simulink model "cordic_test"  (R2020a)
settings: Solver=VariableStepAuto  StartTime=0.0  StopTime=2048*2048  RelTol=1e-3
libraries: library x11, simulink x5, hdlsllib x3, simulink_extras x1
settings Model: SimulationMode=rapid-accelerator  Creator=david  LastModifiedBy=david

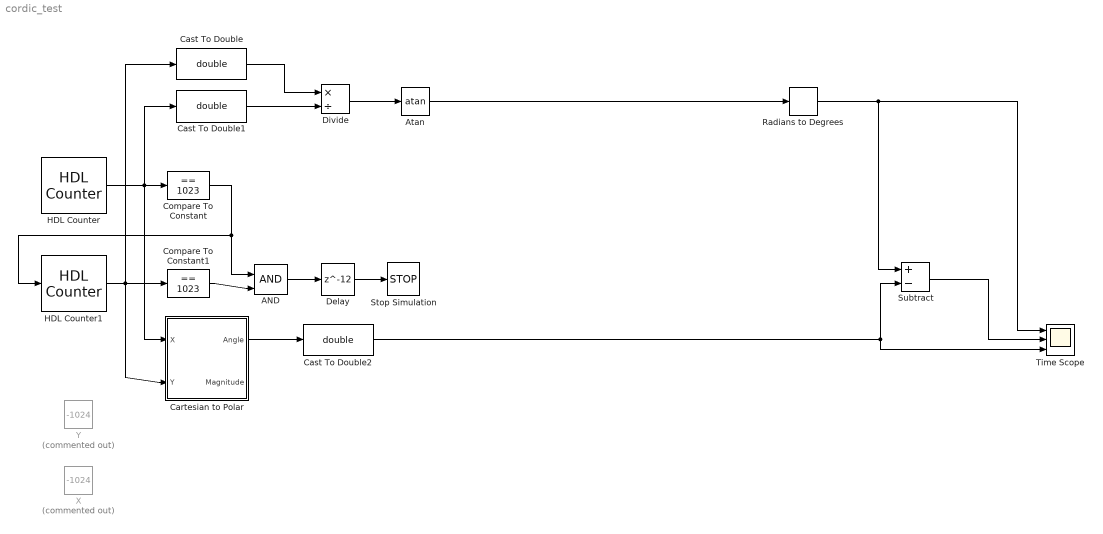
== system cordic_test ==
  AND : Logic  IconShape=distinctive  AllPortsSameDT=off  OutDataTypeStr=boolean
  Atan : Trigonometry  Operator=atan
  Cartesian to Polar : Subsystem  mask{b=16, f=8}
      mask prompts: b "Angle Wordlength:"; f "Angle Fractional Bits:"
      mask DialogControl DescGroupVar Prompt: Cartesian to Polar
      mask DialogControl DescTextVar Prompt: Convert cartesian coordinates to polar representation. This block uses Circular CORDIC operating in vectoring mode. The output angle is in the range [-90, 90] degrees.
      mask DialogControl ParameterGroupVar Prompt: Main
  Cast To Double : DataTypeConversion  OutDataTypeStr=double
  Cast To Double1 : DataTypeConversion  OutDataTypeStr=double
  Cast To Double2 : DataTypeConversion  OutDataTypeStr=double
  Compare To Constant : simulink/Logic and Bit Operations/Compare To Constant  relop===  const=1023  OutDataTypeStr=boolean
  Compare To Constant1 : simulink/Logic and Bit Operations/Compare To Constant  relop===  const=1023  OutDataTypeStr=boolean
  Delay : Delay  DelayLength=12
  Divide : Product  Inputs=*/
  HDL Counter : hdlsllib/Sources/HDL Counter  CountType=Count limited  CountInit=-1024  CountStep=1  CountMax=1023  CountFromType=Initial value  CountFrom=-1024  CountResetPort=off  CountLoadPort=off  CountEnbPort=off  CountDirPort=off  CountDataType=Signed  CountWordLen=24  CountFracLen=11  CountSampTime=1
  HDL Counter1 : hdlsllib/Sources/HDL Counter  CountType=Count limited  CountInit=-1024  CountStep=1  CountMax=1023  CountFromType=Initial value  CountFrom=-1024  CountResetPort=off  CountLoadPort=off  CountEnbPort=on  CountDirPort=off  CountDataType=Signed  CountWordLen=24  CountFracLen=11  CountSampTime=1
  Radians to Degrees : simulink_extras/Transformations/Radians to Degrees
  Stop Simulation : Stop
  Subtract : Sum  Inputs=+-
  Time Scope : Scope  NumInputPorts=3
  X : Constant  Commented=on  Value=-1024  OutDataTypeStr=fixdt(1,16,3)  SampleTime=1
  Y : Constant  Commented=on  Value=-1024  OutDataTypeStr=fixdt(1,16,3)  SampleTime=1
  wires:
  HDL Counter/1 -> Cartesian to Polar/1(X), Cast To Double1/1, Compare To Constant/1
  Compare To Constant/1 -> AND/1, HDL Counter1/1
  Divide/1 -> Atan/1
  HDL Counter1/1 -> Cartesian to Polar/2(Y), Cast To Double/1, Compare To Constant1/1
  Compare To Constant1/1 -> AND/2
  AND/1 -> Delay/1
  Delay/1 -> Stop Simulation/1
  Cast To Double/1 -> Divide/1
  Cast To Double1/1 -> Divide/2
  Atan/1 -> Radians to Degrees/1
  Radians to Degrees/1 -> Subtract/1, Time Scope/1
  Cast To Double2/1 -> Time Scope/3, Subtract/2
  Subtract/1 -> Time Scope/2
  Cartesian to Polar/1(Angle) -> Cast To Double2/1

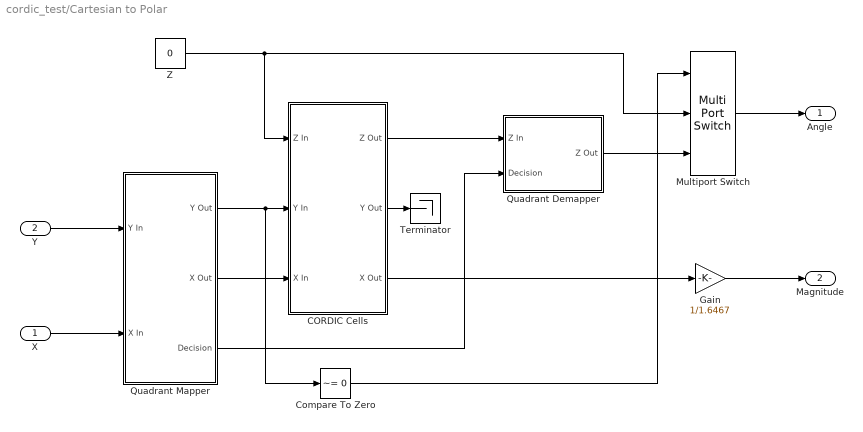
== system cordic_test/Cartesian to Polar ==
  X : Inport
  Y : Inport  Port=2
  CORDIC Cells : Subsystem
  Compare To Zero : simulink/Logic and Bit Operations/Compare To Zero  relop=~=  OutDataTypeStr=boolean
  Gain : Gain  Gain=1/1.6467  ParamDataTypeStr=fixdt(0,16,16)  RndMeth=Round  SaturateOnIntegerOverflow=on  OutDataTypeStr=Inherit: Same as input
  Multiport Switch : MultiPortSwitch  DataPortOrder=Zero-based contiguous  Inputs=2  zeroidx=on
  Quadrant Demapper : Subsystem
  Quadrant Mapper : Subsystem
  Terminator : Terminator
  Z : Constant  Value=0  OutDataTypeStr=fixdt(1,b,f)  SampleTime=1
  Angle : Outport
  Magnitude : Outport  Port=2
  wires:
  Quadrant Mapper/1(Y Out) -> Compare To Zero/1, CORDIC Cells/2(Y In)
  Quadrant Mapper/2(X Out) -> CORDIC Cells/3(X In)
  Z/1 -> Multiport Switch/2, CORDIC Cells/1(Z In)
  CORDIC Cells/3(X Out) -> Gain/1
  CORDIC Cells/2(Y Out) -> Terminator/1
  Quadrant Mapper/3(Decision) -> Quadrant Demapper/2(Decision)
  CORDIC Cells/1(Z Out) -> Quadrant Demapper/1(Z In)
  Compare To Zero/1 -> Multiport Switch/1
  Gain/1 -> Magnitude/1
  X/1 -> Quadrant Mapper/2(X In)
  Y/1 -> Quadrant Mapper/1(Y In)
  Multiport Switch/1 -> Angle/1
  Quadrant Demapper/1(Z Out) -> Multiport Switch/3

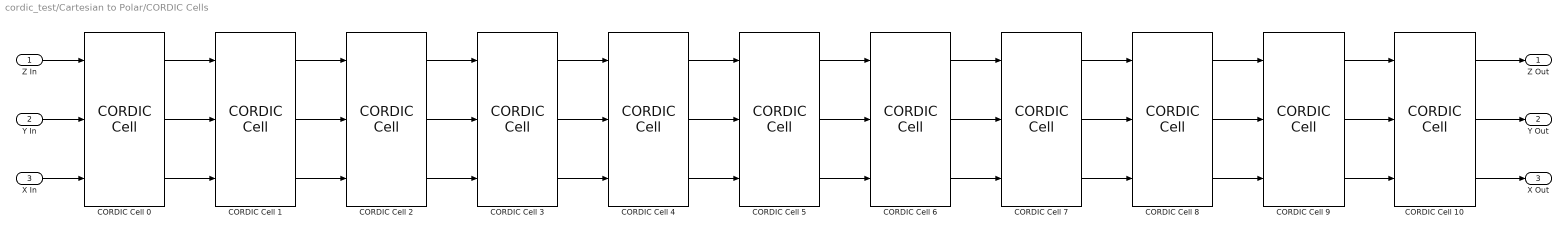
== system cordic_test/Cartesian to Polar/CORDIC Cells ==
  Z In : Inport
  Y In : Inport  Port=2
  X In : Inport  Port=3
  CORDIC Cell 0 : library/CORDIC Cell  k=0
  CORDIC Cell 1 : library/CORDIC Cell  k=1
  CORDIC Cell 10 : library/CORDIC Cell  k=10
  CORDIC Cell 2 : library/CORDIC Cell  k=2
  CORDIC Cell 3 : library/CORDIC Cell  k=3
  CORDIC Cell 4 : library/CORDIC Cell  k=4
  CORDIC Cell 5 : library/CORDIC Cell  k=5
  CORDIC Cell 6 : library/CORDIC Cell  k=6
  CORDIC Cell 7 : library/CORDIC Cell  k=7
  CORDIC Cell 8 : library/CORDIC Cell  k=8
  CORDIC Cell 9 : library/CORDIC Cell  k=9
  Z Out : Outport
  Y Out : Outport  Port=2
  X Out : Outport  Port=3
  wires:
  Y In/1 -> CORDIC Cell 0/2
  X In/1 -> CORDIC Cell 0/3
  Z In/1 -> CORDIC Cell 0/1
  CORDIC Cell 0/2 -> CORDIC Cell 1/2
  CORDIC Cell 0/1 -> CORDIC Cell 1/1
  CORDIC Cell 0/3 -> CORDIC Cell 1/3
  CORDIC Cell 1/3 -> CORDIC Cell 2/3
  CORDIC Cell 1/2 -> CORDIC Cell 2/2
  CORDIC Cell 1/1 -> CORDIC Cell 2/1
  CORDIC Cell 2/2 -> CORDIC Cell 3/2
  CORDIC Cell 2/1 -> CORDIC Cell 3/1
  CORDIC Cell 2/3 -> CORDIC Cell 3/3
  CORDIC Cell 3/2 -> CORDIC Cell 4/2
  CORDIC Cell 3/3 -> CORDIC Cell 4/3
  CORDIC Cell 3/1 -> CORDIC Cell 4/1
  CORDIC Cell 4/2 -> CORDIC Cell 5/2
  CORDIC Cell 4/1 -> CORDIC Cell 5/1
  CORDIC Cell 4/3 -> CORDIC Cell 5/3
  CORDIC Cell 5/2 -> CORDIC Cell 6/2
  CORDIC Cell 5/1 -> CORDIC Cell 6/1
  CORDIC Cell 5/3 -> CORDIC Cell 6/3
  CORDIC Cell 6/3 -> CORDIC Cell 7/3
  CORDIC Cell 6/2 -> CORDIC Cell 7/2
  CORDIC Cell 6/1 -> CORDIC Cell 7/1
  CORDIC Cell 7/3 -> CORDIC Cell 8/3
  CORDIC Cell 7/2 -> CORDIC Cell 8/2
  CORDIC Cell 7/1 -> CORDIC Cell 8/1
  CORDIC Cell 8/2 -> CORDIC Cell 9/2
  CORDIC Cell 8/3 -> CORDIC Cell 9/3
  CORDIC Cell 8/1 -> CORDIC Cell 9/1
  CORDIC Cell 9/2 -> CORDIC Cell 10/2
  CORDIC Cell 9/3 -> CORDIC Cell 10/3
  CORDIC Cell 9/1 -> CORDIC Cell 10/1
  CORDIC Cell 10/1 -> Z Out/1
  CORDIC Cell 10/2 -> Y Out/1
  CORDIC Cell 10/3 -> X Out/1

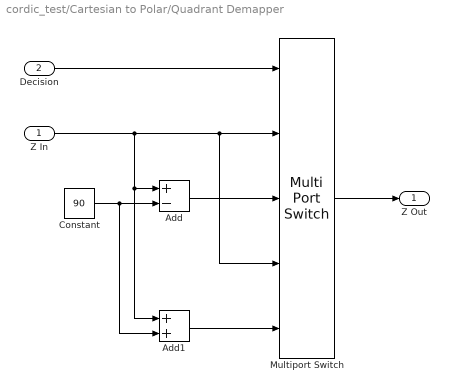
== system cordic_test/Cartesian to Polar/Quadrant Demapper ==
  Z In : Inport
  Decision : Inport  Port=2
  Add : Sum  Inputs=+-  OutDataTypeStr=Inherit: Same as first input
  Add1 : Sum  OutDataTypeStr=Inherit: Same as first input
  Constant : Constant  Value=90  OutDataTypeStr=uint8  SampleTime=-1
  Multiport Switch : MultiPortSwitch  DataPortOrder=Zero-based contiguous  Inputs=4  zeroidx=on
  Z Out : Outport
  wires:
  Decision/1 -> Multiport Switch/1
  Multiport Switch/1 -> Z Out/1
  Z In/1 -> Add1/1, Add/1, Multiport Switch/4, Multiport Switch/2
  Add/1 -> Multiport Switch/3
  Constant/1 -> Add1/2, Add/2
  Add1/1 -> Multiport Switch/5

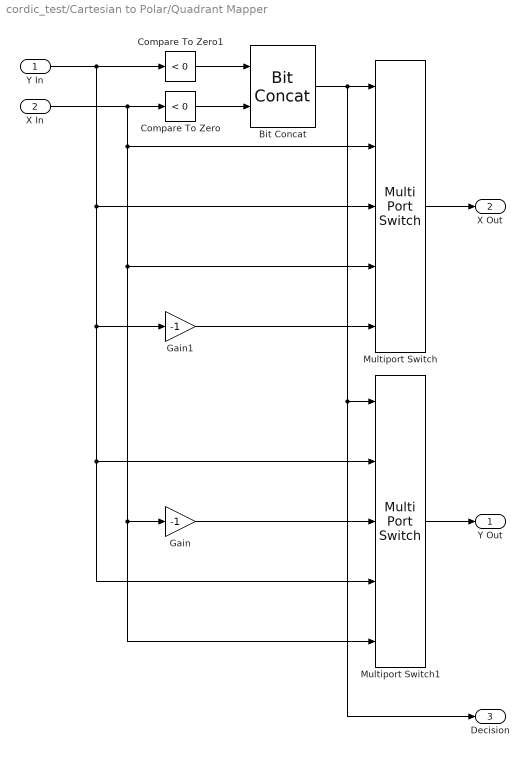
== system cordic_test/Cartesian to Polar/Quadrant Mapper ==
  Y In : Inport
  X In : Inport  Port=2
  Bit Concat : hdlsllib/Logic and Bit Operations/Bit Concat  numInputs=2
  Compare To Zero : simulink/Logic and Bit Operations/Compare To Zero  relop=<  OutDataTypeStr=boolean
  Compare To Zero1 : simulink/Logic and Bit Operations/Compare To Zero  relop=<  OutDataTypeStr=boolean
  Gain : Gain  Gain=-1  OutDataTypeStr=Inherit: Same as input
  Gain1 : Gain  Gain=-1  OutDataTypeStr=Inherit: Same as input
  Multiport Switch : MultiPortSwitch  DataPortOrder=Zero-based contiguous  Inputs=4  zeroidx=on
  Multiport Switch1 : MultiPortSwitch  DataPortOrder=Zero-based contiguous  Inputs=4  zeroidx=on
  Y Out : Outport
  X Out : Outport  Port=2
  Decision : Outport  Port=3
  wires:
  X In/1 -> Compare To Zero/1, Multiport Switch/2, Multiport Switch1/5, Gain/1, Multiport Switch/4
  Compare To Zero1/1 -> Bit Concat/1
  Compare To Zero/1 -> Bit Concat/2
  Bit Concat/1 -> Decision/1, Multiport Switch1/1, Multiport Switch/1
  Multiport Switch/1 -> X Out/1
  Multiport Switch1/1 -> Y Out/1
  Gain/1 -> Multiport Switch1/3
  Gain1/1 -> Multiport Switch/5
  Y In/1 -> Compare To Zero1/1, Multiport Switch/3, Multiport Switch1/2, Multiport Switch1/4, Gain1/1
